simulink model "controlled_fwr_3ph"  (R2024b)
settings: Solver=VariableStepAuto  StartTime=0.0  StopTime=10.0  MaxStep=1e-4  RelTol=1e-3
libraries: spsThyristorLib x12, spsACVoltageSourceLib x6, spsGroundLib x2, spsMeanLib x2, spsSeriesRLCBranchLib x2, spsVoltageMeasurementLib x2, spsCurrentMeasurementLib x1, spsThreePhaseVIMeasurementLib x1, sps_lib x1
settings Model: Creator=Admin  LastModifiedBy=pragy

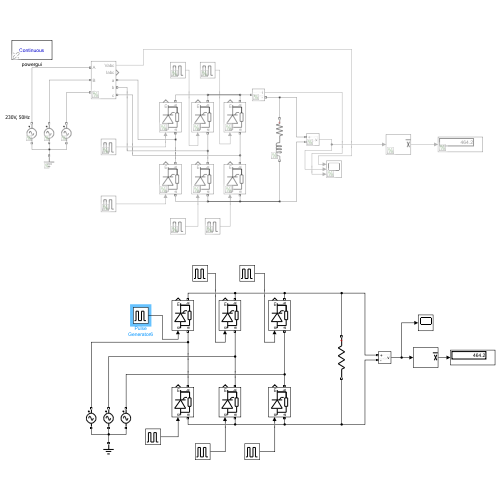
[thumbnail: Simulink's stored preview of the top-level diagram]
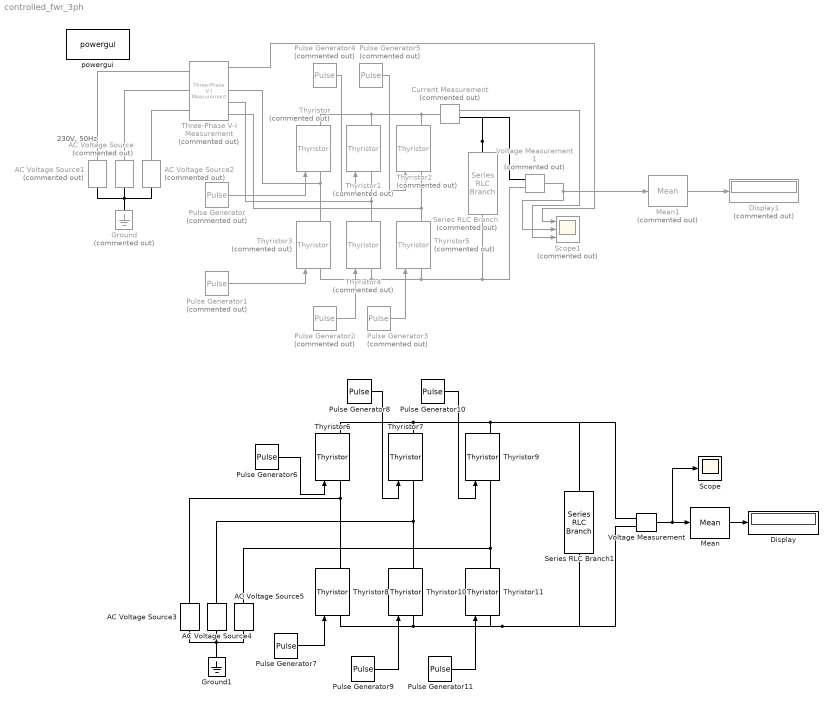
== system controlled_fwr_3ph ==
  note: 230V, 50Hz
  AC Voltage Source : spsACVoltageSourceLib/AC Voltage Source  Commented=on  Amplitude=sqrt(2)*230  Phase=-120  Frequency=50  SampleTime=0  Measurements=None  BusType=swing  Pref=10e3  Qref=0  Qmin=-inf  Qmax=+inf
  AC Voltage Source1 : spsACVoltageSourceLib/AC Voltage Source  Commented=on  Amplitude=sqrt(2)*230  Phase=0  Frequency=50  SampleTime=0  Measurements=None  BusType=swing  Pref=10e3  Qref=0  Qmin=-inf  Qmax=+inf
  AC Voltage Source2 : spsACVoltageSourceLib/AC Voltage Source  Commented=on  Amplitude=sqrt(2)*230  Phase=-240  Frequency=50  SampleTime=0  Measurements=None  BusType=swing  Pref=10e3  Qref=0  Qmin=-inf  Qmax=+inf
  AC Voltage Source3 : spsACVoltageSourceLib/AC Voltage Source  Amplitude=230*sqrt(2)  Phase=0  Frequency=50  SampleTime=0  Measurements=None  BusType=swing  Pref=10e3  Qref=0  Qmin=-inf  Qmax=+inf
  AC Voltage Source4 : spsACVoltageSourceLib/AC Voltage Source  Amplitude=230*sqrt(2)  Phase=-120  Frequency=50  SampleTime=0  Measurements=None  BusType=swing  Pref=10e3  Qref=0  Qmin=-inf  Qmax=+inf
  AC Voltage Source5 : spsACVoltageSourceLib/AC Voltage Source  Amplitude=230*sqrt(2)  Phase=-240  Frequency=50  SampleTime=0  Measurements=None  BusType=swing  Pref=10e3  Qref=0  Qmin=-inf  Qmax=+inf
  Current Measurement : spsCurrentMeasurementLib/Current Measurement  Commented=on  PhasorSimulation=off  OutputType=Complex  PSBequivalent=0
  Display : Display
  Display1 : Display  Commented=on
  Ground : spsGroundLib/Ground  Commented=on  LConnTagsString=a
  Ground1 : spsGroundLib/Ground  LConnTagsString=a
  Mean : spsMeanLib/Mean  Freq=50  Vinit=0  Ts=0
  Mean1 : spsMeanLib/Mean  Commented=on  Freq=50  Vinit=0  Ts=0
  Pulse Generator : DiscretePulseGenerator  Commented=on  PulseType=Time based  Period=0.02  PulseWidth=33.33  PhaseDelay=60*(0.02/360)
  Pulse Generator1 : DiscretePulseGenerator  Commented=on  PulseType=Time based  Period=0.02  PulseWidth=33.33  PhaseDelay=240*(0.02/360)
  Pulse Generator10 : DiscretePulseGenerator  PulseType=Time based  Period=1/50  PulseWidth=33.33  PhaseDelay=(0.02/360)*300
  Pulse Generator11 : DiscretePulseGenerator  PulseType=Time based  Period=1/50  PulseWidth=33.33  PhaseDelay=(0.02/360)*120
  Pulse Generator2 : DiscretePulseGenerator  Commented=on  PulseType=Time based  Period=0.02  PulseWidth=33.33  PhaseDelay=360*(0.02/360)
  Pulse Generator3 : DiscretePulseGenerator  Commented=on  PulseType=Time based  Period=0.02  PulseWidth=33.33  PhaseDelay=120*(0.02/360)
  Pulse Generator4 : DiscretePulseGenerator  Commented=on  PulseType=Time based  Period=0.02  PulseWidth=33.33  PhaseDelay=180*(0.02/360)
  Pulse Generator5 : DiscretePulseGenerator  Commented=on  PulseType=Time based  Period=0.02  PulseWidth=33.33  PhaseDelay=300*(0.02/360)
  Pulse Generator6 : DiscretePulseGenerator  PulseType=Time based  Period=1/50  PulseWidth=33.33  PhaseDelay=(0.02/360)*60
  Pulse Generator7 : DiscretePulseGenerator  PulseType=Time based  Period=1/50  PulseWidth=33.33  PhaseDelay=(0.02/360)*240
  Pulse Generator8 : DiscretePulseGenerator  PulseType=Time based  Period=1/50  PulseWidth=33.33  PhaseDelay=(0.02/360)*180
  Pulse Generator9 : DiscretePulseGenerator  PulseType=Time based  Period=1/50  PulseWidth=33.33  PhaseDelay=(0.02/360)*360
  Scope : Scope
  Scope1 : Scope  Commented=on  NumInputPorts=3
  Series RLC Branch : spsSeriesRLCBranchLib/Series RLC Branch  Commented=on  LConnTagsString=__new0  RConnTagsString=__new0  BranchType=RL  Resistance=10  Inductance=300e-3  SetiL0=off  InitialCurrent=0  Capacitance=1e-6  Setx0=off  InitialVoltage=0  Measurements=None
  Series RLC Branch1 : spsSeriesRLCBranchLib/Series RLC Branch  LConnTagsString=__new0  RConnTagsString=__new0  BranchType=R  Resistance=10  Inductance=1e-3  SetiL0=off  InitialCurrent=0  Capacitance=1e-6  Setx0=off  InitialVoltage=0  Measurements=None
  Three-Phase V-I Measurement : spsThreePhaseVIMeasurementLib/Three-Phase V-I Measurement  Commented=on  VoltageMeasurement=phase-to-ground  SetLabelV=off  LabelV=Vabc  Vpu=off  VpuLL=off  CurrentMeasurement=yes  SetLabelI=off  LabelI=Iabc  Ipu=off  Pbase=100e6  Vbase=500e3  OutputType=Complex  PhasorSimulation=off  PSBequivalent=0
  Thyristor{,1..5} (6 alike) : spsThyristorLib/Thyristor  Commented=on  Ron=0.001  Lon=0  Vf=0.8  IC=0  Rs=500  Cs=250e-9  Measurements=on
  Thyristor{6..11} (6 alike) : spsThyristorLib/Thyristor  Ron=0.001  Lon=0  Vf=0.8  IC=0  Rs=500  Cs=250e-9  Measurements=on
  Voltage Measurement : spsVoltageMeasurementLib/Voltage Measurement  PhasorSimulation=off  OutputType=Complex  PSBequivalent=0
  Voltage Measurement1 : spsVoltageMeasurementLib/Voltage Measurement  Commented=on  PhasorSimulation=off  OutputType=Complex  PSBequivalent=0
  powergui : sps_lib/powergui  Priority=1  SimulationMode=Continuous  SampleTime=50e-6  frequency=60  Iterations=50  frequencyindice=50  Pbase=100e6  ErrMax=1e-4  UnitsV=kV  UnitsW=MW  buscounter=0  FunctionMessages=off  echomessages=off  EnableUseOfTLC=off  CurrentSourceSwitches=off  DisableSnubberDevices=off  DisableRonSwitches=off  DisableVfSwitches=off  DisplayEquations=off  AutomaticDiscreteSolvers=off  SolverType=Tustin/Backward Euler (TBE)  Interpol=off  ExternalGateDelay=off  methode=off  Ts=100  x0status=zero  SPID=on  SwTol=0  HookPort=off  NonlinearTolerance=1e-4  nMaxIteration=100  ContinueOnMaxIteration=off  RestoreLinks=warning  ResistiveCurrentMeasurement=off  Frange=[0:2:500]  Ylog=off  Xlog=on  ShowGrid=off  save=off  variable=ZData  structure=0  ZoomFFT=off  StartTime=0.0  cycles=1  DisplayStyle=1  fundamental=60  FreqAxis=off  MaxFrequency=1000  frequencyindicesteady=1  RmsSteady=1  display=off
  wires:
  Pulse Generator/1 -> Thyristor/1
  Pulse Generator1/1 -> Thyristor3/1
  Pulse Generator2/1 -> Thyristor4/1
  Pulse Generator3/1 -> Thyristor5/1
  Pulse Generator4/1 -> Thyristor1/1
  Pulse Generator5/1 -> Thyristor2/1
  Three-Phase V-I Measurement/1 -> Scope1/1
  Current Measurement/1 -> Scope1/3
  Voltage Measurement1/1 -> Mean1/1, Scope1/2
  Voltage Measurement/1 -> Scope/1, Mean/1
  Mean/1 -> Display/1
  Pulse Generator6/1 -> Thyristor6/1
  Pulse Generator7/1 -> Thyristor8/1
  Pulse Generator8/1 -> Thyristor7/1
  Pulse Generator9/1 -> Thyristor10/1
  Pulse Generator10/1 -> Thyristor9/1
  Pulse Generator11/1 -> Thyristor11/1
  Mean1/1 -> Display1/1
  connections:
  Series RLC Branch/LConn1 -- Voltage Measurement1/LConn1 -- Current Measurement/RConn1
  Voltage Measurement1/LConn2 -- Series RLC Branch/RConn1 -- Thyristor3/LConn1 -- Thyristor4/LConn1 -- Thyristor5/LConn1
  Current Measurement/LConn1 -- Thyristor2/RConn1 -- Thyristor1/RConn1 -- Thyristor/RConn1
  AC Voltage Source/LConn1 -- AC Voltage Source1/LConn1 -- Ground/LConn1 -- AC Voltage Source2/LConn1
  Thyristor5/RConn1 -- Three-Phase V-I Measurement/RConn3 -- Thyristor2/LConn1
  Thyristor1/LConn1 -- Three-Phase V-I Measurement/RConn2 -- Thyristor4/RConn1
  Thyristor3/RConn1 -- Three-Phase V-I Measurement/RConn1 -- Thyristor/LConn1
  AC Voltage Source1/RConn1 -- Three-Phase V-I Measurement/LConn1
  Three-Phase V-I Measurement/LConn2 -- AC Voltage Source/RConn1
  AC Voltage Source2/RConn1 -- Three-Phase V-I Measurement/LConn3
  Thyristor6/RConn1 -- Voltage Measurement/LConn1 -- Series RLC Branch1/LConn1 -- Thyristor9/RConn1 -- Thyristor7/RConn1
  Thyristor6/LConn1 -- AC Voltage Source3/RConn1 -- Thyristor8/RConn1
  Thyristor7/LConn1 -- AC Voltage Source4/RConn1 -- Thyristor10/RConn1
  Thyristor9/LConn1 -- Thyristor11/RConn1 -- AC Voltage Source5/RConn1
  Thyristor8/LConn1 -- Series RLC Branch1/RConn1 -- Voltage Measurement/LConn2 -- Thyristor11/LConn1 -- Thyristor10/LConn1
  AC Voltage Source3/LConn1 -- Ground1/LConn1 -- AC Voltage Source5/LConn1 -- AC Voltage Source4/LConn1
